simulink model "ACC_System"  (R2025b)
settings: Solver=ode4  StartTime=0.0  StopTime=30  FixedStep=0.01  RelTol=1e-3
settings Model: Creator=ghazal  LastModifiedBy=ghazal

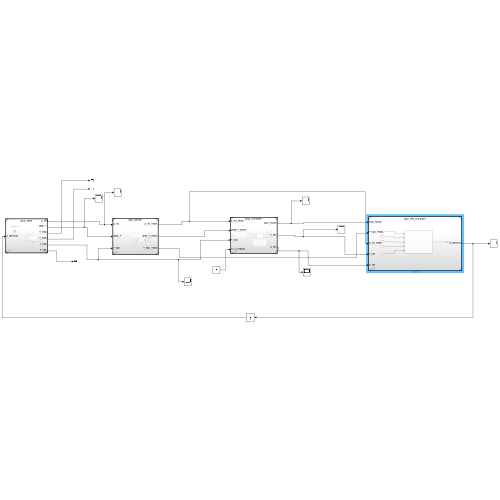
[thumbnail: Simulink's stored preview of the top-level diagram]
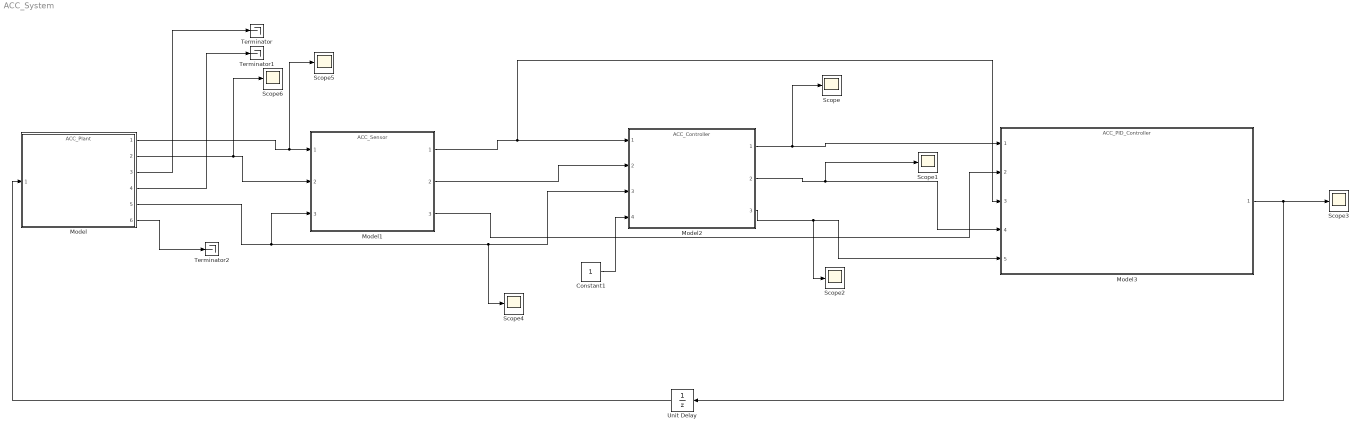
== system ACC_System ==
  Constant1 : Constant
  Model : ModelReference  ModelNameDialog=ACC_Plant.slx  SimulationMode=Normal  ModelReferenceVersion=1.8
  Model1 : ModelReference  ModelNameDialog=ACC_Sensor.slx  SimulationMode=Normal  ModelReferenceVersion=1.15
  Model2 : ModelReference  ModelNameDialog=ACC_Controller.slx  SimulationMode=Normal  ModelReferenceVersion=1.8
  Model3 : ModelReference  ModelNameDialog=ACC_PID_Controller.slx  SimulationMode=Normal  ModelReferenceVersion=1.6
  Scope{,1..6} (7 alike) : Scope
      Scope settings: ActiveDisplayYMinimum=-0.49999999999999989  ActiveDisplayYMaximum=4.5
      Scope1 settings: ActiveDisplayYMinimum=-1  ActiveDisplayYMaximum=1
      Scope2 settings: ActiveDisplayYMinimum=-1  ActiveDisplayYMaximum=1  DataLoggingVariableName=ScopeData2
      Scope3 settings: ActiveDisplayYMinimum=-9.25  ActiveDisplayYMaximum=3.25  DataLoggingVariableName=ScopeData3
      Scope4 settings: ActiveDisplayYMinimum=-4.867951217645671  ActiveDisplayYMaximum=29.847552824035805  DataLoggingVariableName=ScopeData4
      Scope5 settings: ActiveDisplayYMinimum=-1.4483231425669363  ActiveDisplayYMaximum=88.156280105642807  DataLoggingVariableName=ScopeData5
      Scope6 settings: DataLoggingVariableName=ScopeData6
  Terminator : Terminator
  Terminator1 : Terminator
  Terminator2 : Terminator
  Unit Delay : UnitDelay  SampleTime=-1  HasFrameUpgradeWarning=on
  wires:
  Model/1 -> Scope5/1, Model1/1
  Model/2 -> Scope6/1, Model1/2
  Model1/1 -> Model2/1, Model3/3
  Model1/2 -> Model2/2
  Constant1/1 -> Model2/4
  Model/5 -> Model1/3, Scope4/1, Model2/3
  Model2/1 -> Scope/1, Model3/1
  Model2/2 -> Scope1/1, Model3/4
  Model2/3 -> Scope2/1, Model3/5
  Model/3 -> Terminator/1
  Model/4 -> Terminator1/1
  Model/6 -> Terminator2/1
  Model1/3 -> Model3/2
  Model3/1 -> Unit Delay/1, Scope3/1
  Unit Delay/1 -> Model/1
